simulink model "Q7"  (R2016b)
settings: Solver=VariableStepAuto  StartTime=0.0  StopTime=20  RelTol=1e-3
settings Model: Creator=AKSHAY JP PAWAR  LastModifiedBy=AKSHAY JP PAWAR
settings DataIOCC: ReturnWorkspaceOutputs=on
settings SFSimCC: SimUseLocalCustomCode=on
settings RTWCC: RTWUseLocalCustomCode=on

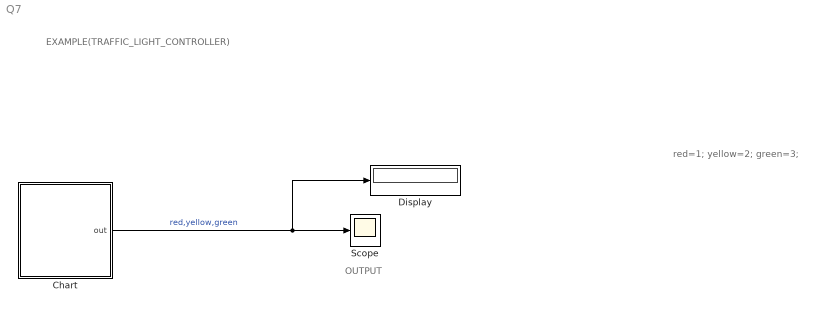
== system Q7 ==
  note: EXAMPLE(TRAFFIC_LIGHT_CONTROLLER)
  note: red=1;
      | yellow=2;
      | green=3;
  note: OUTPUT
  Chart : Stateflow chart  TreatAsAtomicUnit=on
  Display : Display
  Scope : Scope
  wires:
  Chart/1(out) -> Display/1, Scope/1  "red,yellow,green"

== stateflow chart Q7/Chart ==
  state Stop
    entry:
    out=1;
  state Go
    entry:
    out=2;
  state Prepare_stop
    entry:
    out=3;
  (default) -> Stop
  Prepare_stop -> Stop : [after(2,sec)]
  Stop -> Go : [after(2,sec)]
  Go -> Prepare_stop : [after(2,sec)]
  data: out output double
